simulink model "AttitudeFinalProject"  (R2018a)
settings: Solver=VariableStepAuto  StartTime=0.0  StopTime=5000  RelTol=1e-14
settings Model: Creator=computer  LastModifiedBy=computer

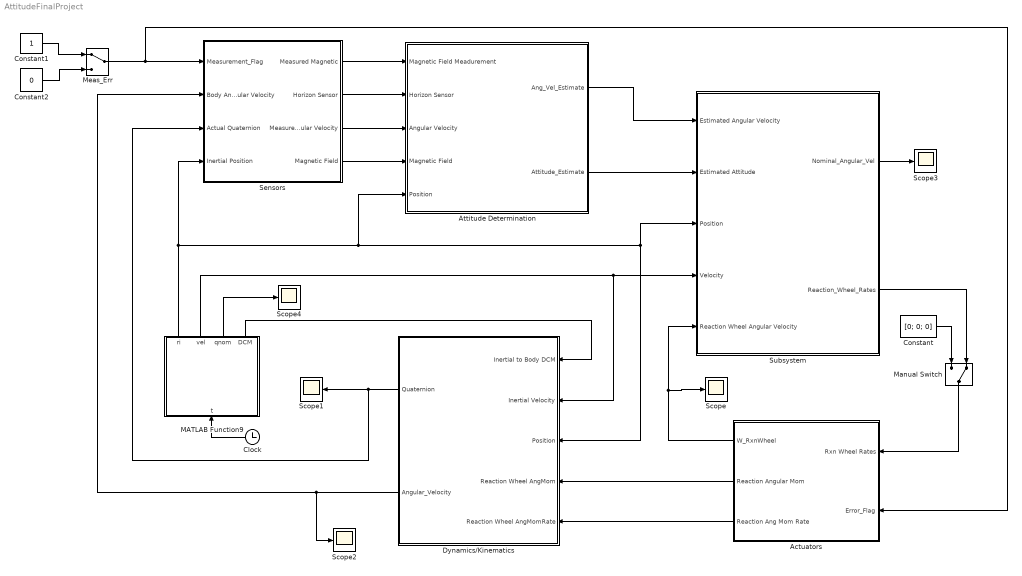
== system AttitudeFinalProject ==
  Actuators : Subsystem
  Attitude Determination : Subsystem
  Clock : Clock
  Constant : Constant  Value=[0; 0; 0]
  Constant1 : Constant
  Constant2 : Constant  Value=0
  Dynamics/Kinematics : Subsystem
  MATLAB Function9 : MATLAB Function  TreatAsAtomicUnit=on
  Manual Switch : ManualSwitch  CurrentSetting=0
  Meas_Err : ManualSwitch
  Scope{,1..4} (5 alike) : Scope
  Sensors : Subsystem
  Subsystem : Subsystem
  wires:
  MATLAB Function9/1(ri) -> Dynamics/Kinematics/3("Position "), Subsystem/3(Position), Attitude Determination/5(Position), Sensors/4(Inertial Position)
  Sensors/3(Measured Angular Velocity) -> Attitude Determination/3(Angular Velocity)
  Sensors/2(Horizon Sensor) -> Attitude Determination/2(Horizon Sensor)
  Sensors/1(Measured Magnetic) -> Attitude Determination/1(Magnetic Field Meadurement)
  Sensors/4(Magnetic Field) -> Attitude Determination/4(Magnetic Field)
  Attitude Determination/1(Ang_Vel_Estimate) -> Subsystem/1(Estimated Angular Velocity)
  Attitude Determination/2(Attitude_Estimate) -> Subsystem/2(Estimated Attitude)
  Subsystem/2(Reaction_Wheel_Rates) -> Manual Switch/2
  Actuators/1(W_RxnWheel) -> Scope/1, Subsystem/5(Reaction Wheel Angular Velocity)
  Actuators/2(Reaction Angular Mom) -> Dynamics/Kinematics/4(Reaction Wheel AngMom)
  Actuators/3(Reaction Ang Mom Rate) -> Dynamics/Kinematics/5("Reaction Wheel AngMomRate ")
  Clock/1 -> MATLAB Function9/1(t)
  Dynamics/Kinematics/1(Quaternion) -> Sensors/3(Actual Quaternion), Scope1/1
  Dynamics/Kinematics/2(Angular_Velocity) -> Sensors/2(Body Angular Velocity), Scope2/1
  MATLAB Function9/2(vel) -> Dynamics/Kinematics/2(Inertial Velocity), Subsystem/4("Velocity ")
  MATLAB Function9/3(qnom) -> Scope4/1
  Constant/1 -> Manual Switch/1
  Manual Switch/1 -> Actuators/1(Rxn Wheel Rates)
  Meas_Err/1 -> Actuators/2("Error_Flag "), Sensors/1("Measurement_Flag ")
  Constant1/1 -> Meas_Err/1
  Constant2/1 -> Meas_Err/2
  MATLAB Function9/4(DCM) -> Dynamics/Kinematics/1("Inertial to Body DCM ")
  Subsystem/1(Nominal_Angular_Vel) -> Scope3/1

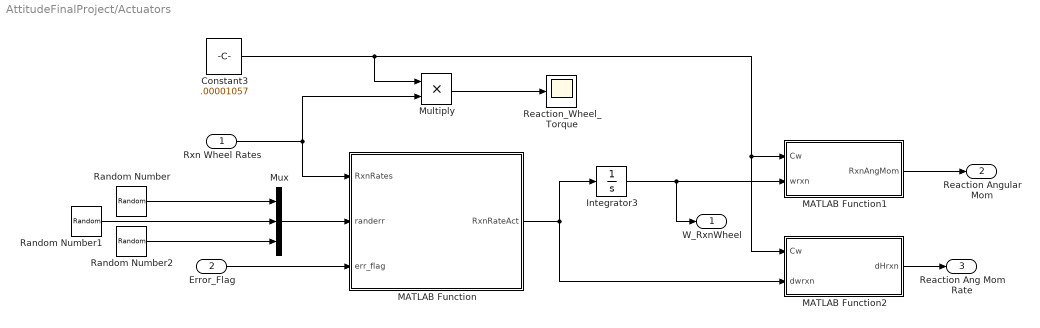
== system AttitudeFinalProject/Actuators ==
  Rxn Wheel Rates : Inport
  "Error_Flag " : Inport  Port=2
  Constant3 : Constant  Value=.00001057
  Integrator3 : Integrator  InitialCondition=[0; 0; 0]
  MATLAB Function : MATLAB Function  TreatAsAtomicUnit=on
  MATLAB Function1 : MATLAB Function  TreatAsAtomicUnit=on
  MATLAB Function2 : MATLAB Function  TreatAsAtomicUnit=on
  Multiply : Product
  Mux : Mux  Inputs=3
  Random Number : RandomNumber  SampleTime=0.1
  Random Number1 : RandomNumber  SampleTime=0.1
  Random Number2 : RandomNumber  SampleTime=0.1
  "Reaction_Wheel_Torque " : Scope
  W_RxnWheel : Outport
  Reaction Angular Mom : Outport  Port=2
  Reaction Ang Mom Rate : Outport  Port=3
  wires:
  Random Number1/1 -> Mux/2
  Random Number/1 -> Mux/1
  Random Number2/1 -> Mux/3
  Mux/1 -> MATLAB Function/2(randerr)
  Rxn Wheel Rates/1 -> MATLAB Function/1(RxnRates), Multiply/2
  MATLAB Function/1(RxnRateAct) -> MATLAB Function2/2(dwrxn), Integrator3/1
  Integrator3/1 -> MATLAB Function1/2(wrxn), W_RxnWheel/1
  MATLAB Function1/1(RxnAngMom) -> Reaction Angular Mom/1
  Constant3/1 -> MATLAB Function2/1(Cw), MATLAB Function1/1(Cw), Multiply/1
  MATLAB Function2/1(dHrxn) -> Reaction Ang Mom Rate/1
  Multiply/1 -> "Reaction_Wheel_Torque "/1
  "Error_Flag "/1 -> MATLAB Function/3(err_flag)

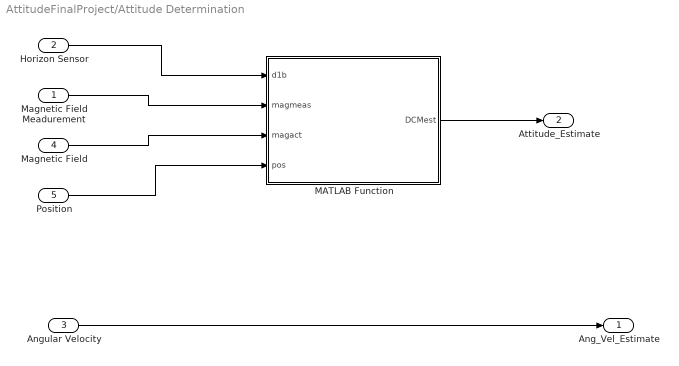
== system AttitudeFinalProject/Attitude Determination ==
  Magnetic Field Meadurement : Inport
  Horizon Sensor : Inport  Port=2
  Angular Velocity : Inport  Port=3
  Magnetic Field : Inport  Port=4
  Position : Inport  Port=5
  MATLAB Function : MATLAB Function  TreatAsAtomicUnit=on
  Ang_Vel_Estimate : Outport
  Attitude_Estimate : Outport  Port=2
  wires:
  Horizon Sensor/1 -> MATLAB Function/1(d1b)
  Position/1 -> MATLAB Function/4(pos)
  Magnetic Field/1 -> MATLAB Function/3(magact)
  Magnetic Field Meadurement/1 -> MATLAB Function/2(magmeas)
  Angular Velocity/1 -> Ang_Vel_Estimate/1
  MATLAB Function/1(DCMest) -> Attitude_Estimate/1

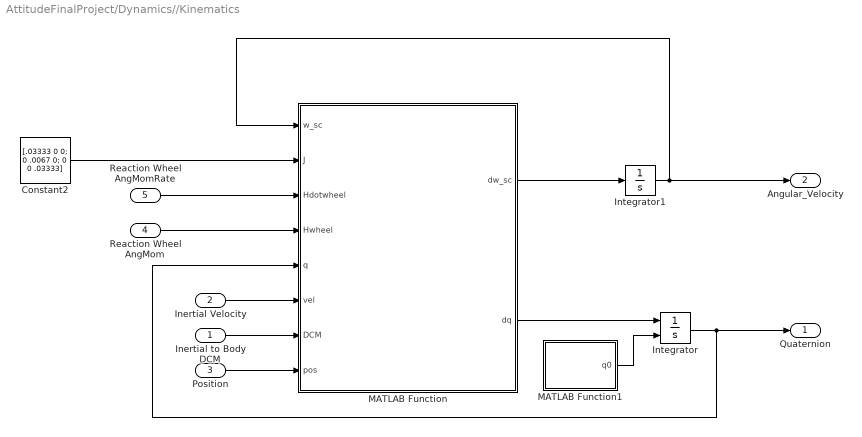
== system AttitudeFinalProject/Dynamics//Kinematics ==
  "Inertial to Body DCM " : Inport
  Inertial Velocity : Inport  Port=2
  "Position " : Inport  Port=3
  Reaction Wheel AngMom : Inport  Port=4
  "Reaction Wheel AngMomRate " : Inport  Port=5
  Constant2 : Constant  Value=[.03333 0 0; 0 .0067 0; 0 0 .03333]
  Integrator : Integrator  InitialConditionSource=external
  Integrator1 : Integrator  InitialCondition=[.005; 0; - sqrt(3.986e14/6600000^3)]
  MATLAB Function : MATLAB Function  TreatAsAtomicUnit=on
  MATLAB Function1 : MATLAB Function  TreatAsAtomicUnit=on
  Quaternion : Outport
  Angular_Velocity : Outport  Port=2
  wires:
  "Reaction Wheel AngMomRate "/1 -> MATLAB Function/3(Hdotwheel)
  Reaction Wheel AngMom/1 -> MATLAB Function/4(Hwheel)
  Constant2/1 -> MATLAB Function/2(J)
  MATLAB Function/2(dq) -> Integrator/1
  Integrator/1 -> Quaternion/1, MATLAB Function/5(q)
  MATLAB Function/1(dw_sc) -> Integrator1/1
  Integrator1/1 -> MATLAB Function/1(w_sc), Angular_Velocity/1
  MATLAB Function1/1(q0) -> Integrator/2
  Inertial Velocity/1 -> MATLAB Function/6(vel)
  "Inertial to Body DCM "/1 -> MATLAB Function/7(DCM)
  "Position "/1 -> MATLAB Function/8(pos)

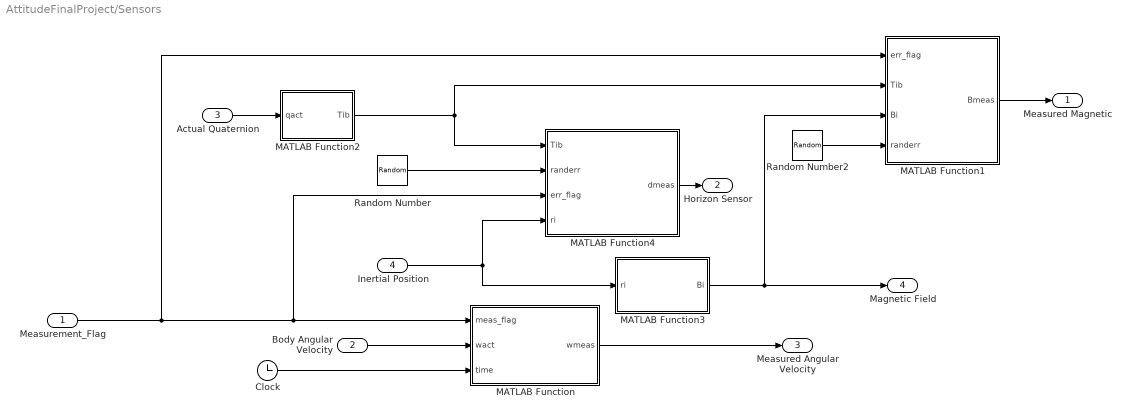
== system AttitudeFinalProject/Sensors ==
  "Measurement_Flag " : Inport
  Body Angular Velocity : Inport  Port=2
  Actual Quaternion : Inport  Port=3
  Inertial Position : Inport  Port=4
  Clock : Clock
  MATLAB Function : MATLAB Function  TreatAsAtomicUnit=on
  MATLAB Function1 : MATLAB Function  TreatAsAtomicUnit=on
  MATLAB Function2 : MATLAB Function  TreatAsAtomicUnit=on
  MATLAB Function3 : MATLAB Function  TreatAsAtomicUnit=on
  MATLAB Function4 : MATLAB Function  TreatAsAtomicUnit=on
  Random Number : RandomNumber  Mean=zeros(3)  Variance=ones(3)  Seed=[0 1 2; 3 4 5; 6 7 8]  SampleTime=0.1
  Random Number2 : RandomNumber  Mean=[0; 0; 0]  Variance=[1; 1; 1]  Seed=[1; 3; 5]  SampleTime=0.1
  Measured Magnetic : Outport
  Horizon Sensor : Outport  Port=2
  Measured Angular Velocity : Outport  Port=3
  Magnetic Field : Outport  Port=4
  wires:
  Body Angular Velocity/1 -> MATLAB Function/2(wact)
  MATLAB Function2/1(Tib) -> MATLAB Function1/2(Tib), MATLAB Function4/1(Tib)
  Inertial Position/1 -> MATLAB Function4/4(ri), MATLAB Function3/1(ri)
  MATLAB Function3/1(Bi) -> MATLAB Function1/3(Bi), Magnetic Field/1
  Actual Quaternion/1 -> MATLAB Function2/1(qact)
  MATLAB Function/1(wmeas) -> Measured Angular Velocity/1
  MATLAB Function4/1(dmeas) -> Horizon Sensor/1
  Random Number/1 -> MATLAB Function4/2(randerr)
  MATLAB Function1/1(Bmeas) -> Measured Magnetic/1
  Clock/1 -> MATLAB Function/3(time)
  Random Number2/1 -> MATLAB Function1/4(randerr)
  "Measurement_Flag "/1 -> MATLAB Function4/3(err_flag), MATLAB Function/1(meas_flag), MATLAB Function1/1(err_flag)

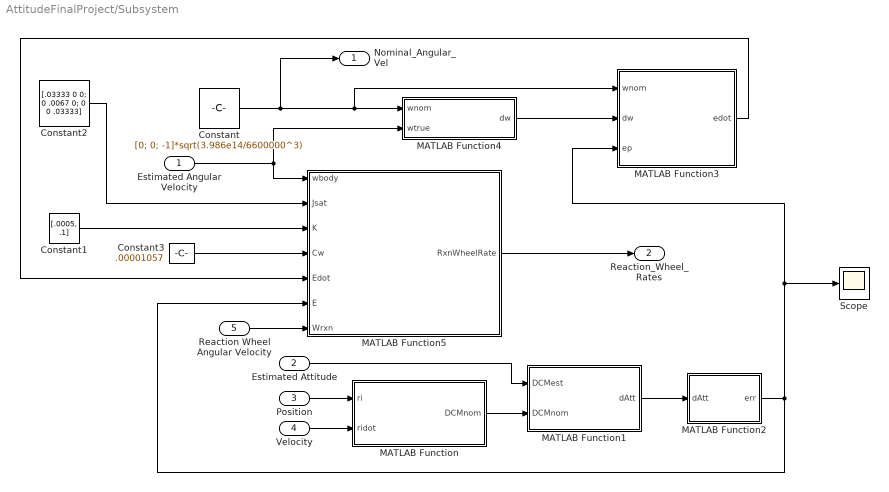
== system AttitudeFinalProject/Subsystem ==
  Estimated Angular Velocity : Inport
  Estimated Attitude : Inport  Port=2
  Position : Inport  Port=3
  "Velocity " : Inport  Port=4
  Reaction Wheel Angular Velocity : Inport  Port=5
  Constant : Constant  Value=[0; 0; -1]*sqrt(3.986e14/6600000^3)
  Constant1 : Constant  Value=[.0005, .1]
  Constant2 : Constant  Value=[.03333 0 0; 0 .0067 0; 0 0 .03333]
  Constant3 : Constant  Value=.00001057
  MATLAB Function : MATLAB Function  TreatAsAtomicUnit=on
  MATLAB Function1 : MATLAB Function  TreatAsAtomicUnit=on
  MATLAB Function2 : MATLAB Function  TreatAsAtomicUnit=on
  MATLAB Function3 : MATLAB Function  TreatAsAtomicUnit=on
  MATLAB Function4 : MATLAB Function  TreatAsAtomicUnit=on
  MATLAB Function5 : MATLAB Function  TreatAsAtomicUnit=on
  Scope : Scope
  Nominal_Angular_Vel : Outport
  Reaction_Wheel_Rates : Outport  Port=2
  wires:
  Position/1 -> MATLAB Function/1(ri)
  "Velocity "/1 -> MATLAB Function/2(ridot)
  MATLAB Function/1(DCMnom) -> MATLAB Function1/2(DCMnom)
  Estimated Attitude/1 -> MATLAB Function1/1(DCMest)
  MATLAB Function1/1(dAtt) -> MATLAB Function2/1(dAtt)
  MATLAB Function2/1(err) -> Scope/1, MATLAB Function3/3(ep), MATLAB Function5/6(E)
  Estimated Angular Velocity/1 -> MATLAB Function5/1(wbody), MATLAB Function4/2(wtrue)
  MATLAB Function4/1(dw) -> MATLAB Function3/2(dw)
  Constant/1 -> Nominal_Angular_Vel/1, MATLAB Function3/1(wnom), MATLAB Function4/1(wnom)
  MATLAB Function3/1(edot) -> MATLAB Function5/5(Edot)
  MATLAB Function5/1(RxnWheelRate) -> Reaction_Wheel_Rates/1
  Constant2/1 -> MATLAB Function5/2(Jsat)
  Constant1/1 -> MATLAB Function5/3(K)
  Reaction Wheel Angular Velocity/1 -> MATLAB Function5/7(Wrxn)
  Constant3/1 -> MATLAB Function5/4(Cw)

== matlab function AttitudeFinalProject/Dynamics//Kinematics/MATLAB Function1 ==
  data: q0 output
function q0 = fcn()
p = 6657000;   % m
mu = 3.986e14; % m^3/s^2
w = sqrt(mu/p^3);

ri = (p/sqrt(2))*[-cos(0); sqrt(2)*sin(0); cos(0)];
bx = -ri/norm(ri);

ridot = (w*p/sqrt(2))*[sin(0); sqrt(2)*cos(0); -sin(0)];
by = ridot/norm(ridot);

bz = cross(bx, by);

DCM = [bx'; by'; bz'];

qs = .5*sqrt(1 + trace(DCM));
qx = (DCM(3,2) - DCM(2,3))/(4*qs);
qy = (DCM(1,3) - DCM(3,1))/(4*qs);
qz = (DCM(2,1) - DCM(1,2))/(4*qs);

q0nom = [qx; qy; qz; qs];

thetaerr = 2;
qerr = [0; sind(thetaerr/2); 0; cosd(thetaerr/2)];

q0 = qmult(qerr, q0nom);

== matlab function AttitudeFinalProject/MATLAB Function9 ==
  data: ri output; vel output; t input; qnom output; DCM output
function [ri, vel, qnom, DCM] = Pos_Vel(t)

p = 6657000;   % m
mu = 3.986e14; % m^3/s^2
w = sqrt(mu/p^3);

ri = (p/sqrt(2))*[-cos(w*t); sqrt(2)*sin(w*t); cos(w*t)];
bx = -ri/norm(ri);

ridot = (w*p/sqrt(2))*[sin(w*t); sqrt(2)*cos(w*t); -sin(w*t)];
by = ridot/norm(ridot);

bz = cross(bx, by);

DCM = [bx'; by'; bz'];

qs = .5*sqrt(1 + trace(DCM))*sign(DCM(2,1));
qx = (DCM(2,3) - DCM(3,2))/(4*qs);
qy = (DCM(3,1) - DCM(1,3))/(4*qs);
qz = (DCM(1,2) - DCM(2,1))/(4*qs);

qnom = [qx; qy; qz; qs]; % inertial to body quaternion - scalar part last

vel = ridot;

== matlab function AttitudeFinalProject/Attitude Determination/MATLAB Function ==
  data: d1b input; magmeas input; magact input; DCMest output; pos input
function DCMest = TRIAD(d1b, magmeas, magact, pos)

d1i = -pos/norm(pos);
d2i = magact/norm(magact);

d2b = magmeas/norm(magmeas);


xb = d1b;
yb = cross(d1b, d2b)/norm(cross(d1b, d2b));
zb = cross(xb, yb);

xi = d1i;
yi = cross(d1i, d2i)/norm(cross(d1i, d2i));
zi = cross(xi, yi);

DCMest = [xb yb zb]*[xi yi zi]';

== matlab function AttitudeFinalProject/Sensors/MATLAB Function ==
  data: meas_flag input; wact input; wmeas output; time input
function wmeas = Measure_Ang_Vel(meas_flag, wact, time)

b = 1;             % gyro bias deg/hr

b = b*pi/180/3600; % gyro bias rad/s

gyro_walk = .22;     % angular random walk vgyro(t)
                      % deg/hr

vgyro = (gyro_walk*(pi/180)/(60))^2; % rad/s

gyro_walk_randomize = [.8147; .9058; .1270]; 
% constants from MATLAB rand to ensure non-uniform walk in 
% each direction
perturbations = b + vgyro*time*gyro_walk_randomize;

if ~meas_flag
    perturbations = [0; 0; 0];
end

wmeas = wact + perturbations;

== matlab function AttitudeFinalProject/Sensors/MATLAB Function1 ==
  data: err_flag input; Tib input; Bi input; Bmeas output; randerr input
function Bmeas = mag_measure(err_flag, Tib, Bi, randerr)

vmag = 0;

if err_flag
    vmag = 8e-9;  % magnetomer error vmag(t)
end


Bmeas = Tib*Bi + vmag*randerr;

== matlab function AttitudeFinalProject/Sensors/MATLAB Function2 ==
  data: qact input; Tib output
function Tib = DCM(qact)

qv = qact(1:3);

qvx = [0 -qv(3) qv(2);
    qv(3) 0 -qv(1);
    -qv(2) qv(1) 0];

Tib = eye(3) - 2*qact(4)*qvx + 2*qvx*qvx;

== matlab function AttitudeFinalProject/Sensors/MATLAB Function3 ==
  data: ri input; Bi output
function Bi = Magnetic_Field(ri)

Bo = 3.12e-5;
Re = 6378000;

nz2i = -ri/norm(ri);
ny2i = cross(nz2i, [1; 0; 0])/norm(cross(nz2i, [1; 0; 0]));
nx2i = cross(ny2i, nz2i);
Ti2n = [nx2i'; ny2i'; nz2i'];

rxy = sqrt(ri(1)^2 + ri(2)^2);

lat = atan2(ri(3), rxy);

Bn = Bo*(Re/norm(ri))^3*[cos(lat); 0; -2*sin(lat)];

Bi = (Ti2n')*Bn;

== matlab function AttitudeFinalProject/Sensors/MATLAB Function4 ==
  data: Tib input; randerr input; err_flag input; dmeas output; ri input
function dmeas = Horizon_Sensor(Tib, randerr, err_flag, ri)

horizon_sensor_err = 1; %deg
scale = horizon_sensor_err*pi/180;

if ~err_flag
    scale = 0;
end

Trand = eye(3) - scale*randerr;  % horizon error vhor -> random 3x3 err mat

dmeas = Trand*Tib*(-ri/norm(ri));

== matlab function AttitudeFinalProject/Subsystem/MATLAB Function ==
  data: ri input; DCMnom output; ridot input
function DCMnom = Nominal_Attitude(ri, ridot)

bx = -ri/norm(ri);

by = ridot/norm(ridot);

bz = cross(bx, by);

DCMnom = [bx'; by'; bz'];

== matlab function AttitudeFinalProject/Subsystem/MATLAB Function1 ==
  data: DCMest input; DCMnom input; dAtt output
function dAtt = dAtt(DCMest, DCMnom)

dAtt = DCMest*DCMnom';

== matlab function AttitudeFinalProject/Subsystem/MATLAB Function2 ==
  data: dAtt input; err output
function err = Error(dAtt)

err = -.5*[dAtt(3,2) - dAtt(2,3);
    dAtt(1,3) - dAtt(3,1);
    dAtt(2,1) - dAtt(1,2)];

== matlab function AttitudeFinalProject/Subsystem/MATLAB Function3 ==
  data: wnom input; edot output; dw input; ep input
function edot = errdot(wnom, dw, ep)

wx = wnom(1); wy = wnom(2); wz = wnom(3);
wnomcross = [0 -wz wy;
    wz 0 -wx;
    -wy wx 0];

edot = -wnomcross*ep + dw;

== matlab function AttitudeFinalProject/Subsystem/MATLAB Function4 ==
  data: wnom input; wtrue input; dw output
function dw = werr(wnom, wtrue)

dw = wtrue - wnom;

== matlab function AttitudeFinalProject/Subsystem/MATLAB Function5 ==
  data: wbody input; Jsat input; RxnWheelRate output; K input; Cw input; Edot input; E input; Wrxn input
function RxnWheelRate = Rxn_Wheel_Rates(wbody, Jsat, K, Cw, Edot, E, Wrxn)

RxnWheelRate = Jsat*K(1)*E/Cw + Jsat*K(2)*Edot/Cw - cross(wbody, Wrxn);

== matlab function AttitudeFinalProject/Actuators/MATLAB Function ==
  data: RxnRateAct output; RxnRates input; randerr input; err_flag input
function RxnRateAct = Rxn_Rates_Actual(RxnRates, randerr, err_flag)

Rpm_Max = 10000;
reaction_wheel_error = 5; % +- reaction wheel rpm error
w_Percent_Err = reaction_wheel_error/Rpm_Max;
pert = w_Percent_Err*randerr*norm(RxnRates);

if ~err_flag
    pert = [0; 0; 0];
end

RxnRateAct = RxnRates + pert;

== matlab function AttitudeFinalProject/Actuators/MATLAB Function1 ==
  data: Cw input; wrxn input; RxnAngMom output
function RxnAngMom = Rxn_Ang_Mom(Cw, wrxn)

RxnAngMom = Cw*wrxn;

== matlab function AttitudeFinalProject/Actuators/MATLAB Function2 ==
  data: Cw input; dwrxn input; dHrxn output
function dHrxn = AngMomRate(Cw, dwrxn)

dHrxn = Cw*dwrxn;

== matlab function AttitudeFinalProject/Dynamics//Kinematics/MATLAB Function ==
  data: w_sc input; J input; dw_sc output; Hdotwheel input; Hwheel input; q input; dq output; vel input; DCM input; pos input
function [dw_sc, dq] = ...
ang_accel(w_sc, J, Hdotwheel, Hwheel, q, vel, DCM, pos)

% === Aerodynamic TOrque Perturbation === %
A = .1*.1; % m^2
Cd = 4;
p = 2e-11; %kg/m^3
vhat = vel/norm(vel);
Fd = -.5*p*dot(vel, vel)*Cd*A*DCM*vhat*dot(vhat, [0 1 0]);

r_cg = [.01; .15; .01]; % 3u cubesat

Maero = cross(r_cg, Fd);

% === Gravity Gradient Perturbation === %

GM = 3.986e14;
r = norm(pos);
Mgrav = 3*GM*cross(pos, J*pos)/(r^5);



dw_sc = J\(cross(w_sc, J*w_sc) - Hdotwheel ...
 - cross(w_sc, Hwheel) + Maero + Mgrav);

wq = [w_sc(1); w_sc(2); w_sc(3); 0];

dq = .5*qmult(wq, q);
